simulink library "sm_flex_body_lib"  (R2016b)
settings: Solver=VariableStepAuto  StartTime=0.0  StopTime=10.0  RelTol=1e-3
values from neighbouring files (symbols this model uses):
  frameBody = splitBodyProps    [sm_flex_body_lib_fei_configure_beam.m]
undefined symbols (not defined in the file or in its folder): frameGraphic, X, Y, Z
undefined symbols (not defined in the file): beam_color, beam_opacity, beam_wall, beam_width, beamLink, brot_beamx, brot_beamy, brot_beamz, btra_beamx, elem_length, Extr_Data_Box, krot_beamx, krot_beamy, krot_beamz, ktra_beamx, rho, tau
libraries: sm_flex_body_lib x26, sm_lib x25, nesl_utility x24
(part 2 of 2)

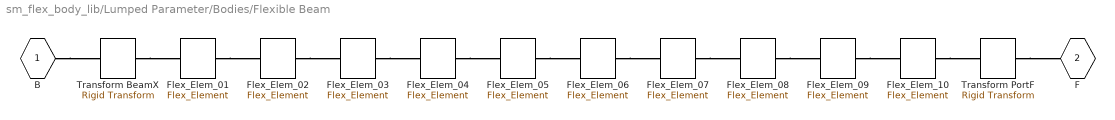
== system sm_flex_body_lib/Lumped Parameter/Bodies/Flexible Beam ==
  Flex_Elem_01 : sm_flex_body_lib/Lumped Parameter/Bodies/Flex_Element  be_length=elem_length  rho=rho  be_color=beam_color  be_opacity=beam_opacity  krot_beamz_elem=krot_beamz  brot_beamz_elem=brot_beamz  krot_beamy_elem=krot_beamy  brot_beamy_elem=brot_beamy  krot_beamx_elem=krot_beamx  brot_beamx_elem=brot_beamx  ktra_beamx_elem=ktra_beamx  btra_beamx_elem=btra_beamx  radio_flextype_elem=Rotation: Z
  Flex_Elem_02 : sm_flex_body_lib/Lumped Parameter/Bodies/Flex_Element  be_length=elem_length  rho=rho  be_color=beam_color  be_opacity=beam_opacity  krot_beamz_elem=krot_beamz  brot_beamz_elem=brot_beamz  krot_beamy_elem=krot_beamy  brot_beamy_elem=brot_beamy  krot_beamx_elem=krot_beamx  brot_beamx_elem=brot_beamx  ktra_beamx_elem=ktra_beamx  btra_beamx_elem=btra_beamx  radio_flextype_elem=Rotation: Z
  Flex_Elem_03 : sm_flex_body_lib/Lumped Parameter/Bodies/Flex_Element  be_length=elem_length  rho=rho  be_color=beam_color  be_opacity=beam_opacity  krot_beamz_elem=krot_beamz  brot_beamz_elem=brot_beamz  krot_beamy_elem=krot_beamy  brot_beamy_elem=brot_beamy  krot_beamx_elem=krot_beamx  brot_beamx_elem=brot_beamx  ktra_beamx_elem=ktra_beamx  btra_beamx_elem=btra_beamx  radio_flextype_elem=Rotation: Z
  Flex_Elem_04 : sm_flex_body_lib/Lumped Parameter/Bodies/Flex_Element  be_length=elem_length  rho=rho  be_color=beam_color  be_opacity=beam_opacity  krot_beamz_elem=krot_beamz  brot_beamz_elem=brot_beamz  krot_beamy_elem=krot_beamy  brot_beamy_elem=brot_beamy  krot_beamx_elem=krot_beamx  brot_beamx_elem=brot_beamx  ktra_beamx_elem=ktra_beamx  btra_beamx_elem=btra_beamx  radio_flextype_elem=Rotation: Z
  Flex_Elem_05 : sm_flex_body_lib/Lumped Parameter/Bodies/Flex_Element  be_length=elem_length  rho=rho  be_color=beam_color  be_opacity=beam_opacity  krot_beamz_elem=krot_beamz  brot_beamz_elem=brot_beamz  krot_beamy_elem=krot_beamy  brot_beamy_elem=brot_beamy  krot_beamx_elem=krot_beamx  brot_beamx_elem=brot_beamx  ktra_beamx_elem=ktra_beamx  btra_beamx_elem=btra_beamx  radio_flextype_elem=Rotation: Z
  Flex_Elem_06 : sm_flex_body_lib/Lumped Parameter/Bodies/Flex_Element  be_length=elem_length  rho=rho  be_color=beam_color  be_opacity=beam_opacity  krot_beamz_elem=krot_beamz  brot_beamz_elem=brot_beamz  krot_beamy_elem=krot_beamy  brot_beamy_elem=brot_beamy  krot_beamx_elem=krot_beamx  brot_beamx_elem=brot_beamx  ktra_beamx_elem=ktra_beamx  btra_beamx_elem=btra_beamx  radio_flextype_elem=Rotation: Z
  Flex_Elem_07 : sm_flex_body_lib/Lumped Parameter/Bodies/Flex_Element  be_length=elem_length  rho=rho  be_color=beam_color  be_opacity=beam_opacity  krot_beamz_elem=krot_beamz  brot_beamz_elem=brot_beamz  krot_beamy_elem=krot_beamy  brot_beamy_elem=brot_beamy  krot_beamx_elem=krot_beamx  brot_beamx_elem=brot_beamx  ktra_beamx_elem=ktra_beamx  btra_beamx_elem=btra_beamx  radio_flextype_elem=Rotation: Z
  Flex_Elem_08 : sm_flex_body_lib/Lumped Parameter/Bodies/Flex_Element  be_length=elem_length  rho=rho  be_color=beam_color  be_opacity=beam_opacity  krot_beamz_elem=krot_beamz  brot_beamz_elem=brot_beamz  krot_beamy_elem=krot_beamy  brot_beamy_elem=brot_beamy  krot_beamx_elem=krot_beamx  brot_beamx_elem=brot_beamx  ktra_beamx_elem=ktra_beamx  btra_beamx_elem=btra_beamx  radio_flextype_elem=Rotation: Z
  Flex_Elem_09 : sm_flex_body_lib/Lumped Parameter/Bodies/Flex_Element  be_length=elem_length  rho=rho  be_color=beam_color  be_opacity=beam_opacity  krot_beamz_elem=krot_beamz  brot_beamz_elem=brot_beamz  krot_beamy_elem=krot_beamy  brot_beamy_elem=brot_beamy  krot_beamx_elem=krot_beamx  brot_beamx_elem=brot_beamx  ktra_beamx_elem=ktra_beamx  btra_beamx_elem=btra_beamx  radio_flextype_elem=Rotation: Z
  Flex_Elem_10 : sm_flex_body_lib/Lumped Parameter/Bodies/Flex_Element  be_length=elem_length  rho=rho  be_color=beam_color  be_opacity=beam_opacity  krot_beamz_elem=krot_beamz  brot_beamz_elem=brot_beamz  krot_beamy_elem=krot_beamy  brot_beamy_elem=brot_beamy  krot_beamx_elem=krot_beamx  brot_beamx_elem=brot_beamx  ktra_beamx_elem=ktra_beamx  btra_beamx_elem=btra_beamx  radio_flextype_elem=Rotation: Z
  Transform BeamX : sm_lib/Frames and Transforms/Rigid Transform  TranslationMethod=StandardAxis  TranslationStandardOffset=0  TranslationLengthUnit=m  TranslationStandardAxis=+Z  TranslationCartesianOffset=[0 0 0]  TranslationROffset=0  TranslationROffsetUnits=m  TranslationZOffset=0  TranslationZOffsetUnits=m  TranslationThetaOffset=0  TranslationThetaOffsetUnits=deg  RotationMethod=StandardAxis  RotationAngleUnits=deg  RotationStandardAxis=+Y  RotationAngle=90  RotationArbitraryAxis=[0 0 1]  FollAlignAxisA=+X  BaseAlignAxisA=+Y  FollAlignAxisB=+Y  BaseAlignAxisB=+Z  RotationSequenceAxes=FollowerAxes  RotationSequence=XYX  RotationSequenceAngles=[0 0 0]  RotationSequenceAnglesUnits=deg  RotationMatrix=[1 0 0; 0 1 0; 0 0 1]
  Transform PortF : sm_lib/Frames and Transforms/Rigid Transform  TranslationMethod=None  TranslationStandardOffset=0  TranslationLengthUnit=m  TranslationStandardAxis=+Z  TranslationCartesianOffset=[0 0 0]  TranslationROffset=0  TranslationROffsetUnits=m  TranslationZOffset=0  TranslationZOffsetUnits=m  TranslationThetaOffset=0  TranslationThetaOffsetUnits=deg  RotationMethod=StandardAxis  RotationAngleUnits=deg  RotationStandardAxis=+Y  RotationAngle=-90  RotationArbitraryAxis=[0 0 1]  FollAlignAxisA=+X  BaseAlignAxisA=+Y  FollAlignAxisB=+Y  BaseAlignAxisB=+Z  RotationSequenceAxes=FollowerAxes  RotationSequence=XYX  RotationSequenceAngles=[0 0 0]  RotationSequenceAnglesUnits=deg  RotationMatrix=[1 0 0; 0 1 0; 0 0 1]
  B : PMIOPort  Port=1  Side=Left
  F : PMIOPort  Port=2  Side=Right
  connections:
  B/RConn1 -- Transform BeamX/LConn1
  Transform BeamX/RConn1 -- Flex_Elem_01/LConn1
  Flex_Elem_01/RConn1 -- Flex_Elem_02/LConn1
  Flex_Elem_02/RConn1 -- Flex_Elem_03/LConn1
  Flex_Elem_03/RConn1 -- Flex_Elem_04/LConn1
  Flex_Elem_04/RConn1 -- Flex_Elem_05/LConn1
  Flex_Elem_05/RConn1 -- Flex_Elem_06/LConn1
  Flex_Elem_06/RConn1 -- Flex_Elem_07/LConn1
  Flex_Elem_07/RConn1 -- Flex_Elem_08/LConn1
  Flex_Elem_08/RConn1 -- Flex_Elem_09/LConn1
  Flex_Elem_09/RConn1 -- Flex_Elem_10/LConn1
  Flex_Elem_10/RConn1 -- Transform PortF/LConn1
  Transform PortF/RConn1 -- F/RConn1

== system sm_flex_body_lib/FE Import/Bodies/Body 3 Frames/Routing Forces ==
  In1 : Inport
  Demux : Demux  Outputs=6*ones(1,3)
  F1 : Outport
  F2 : Outport  Port=2
  F3 : Outport  Port=3
  wires:
  Demux/2 -> F2/1
  In1/1 -> Demux/1
  Demux/1 -> F1/1
  Demux/3 -> F3/1

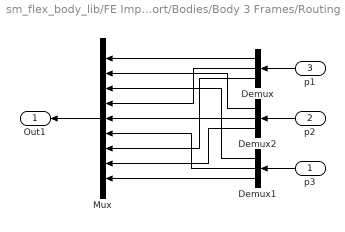
== system sm_flex_body_lib/FE Import/Bodies/Body 3 Frames/Routing pva ==
  p3 : Inport
  p2 : Inport  Port=2
  p1 : Inport  Port=3
  Demux : Demux  Outputs=3
  Demux1 : Demux  Outputs=3
  Demux2 : Demux  Outputs=3
  Mux : Mux  Inputs=9
  Out1 : Outport
  wires:
  Demux2/1 -> Mux/2
  Demux2/2 -> Mux/5
  Demux2/3 -> Mux/8
  p2/1 -> Demux2/1
  Demux1/3 -> Mux/9
  Demux/3 -> Mux/7
  Demux1/2 -> Mux/6
  Demux/2 -> Mux/4
  Demux1/1 -> Mux/3
  Demux/1 -> Mux/1
  p3/1 -> Demux1/1
  Mux/1 -> Out1/1
  p1/1 -> Demux/1

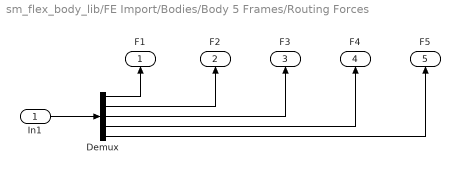
== system sm_flex_body_lib/FE Import/Bodies/Body 5 Frames/Routing Forces ==
  In1 : Inport
  Demux : Demux  Outputs=6*ones(1,5)
  F1 : Outport
  F2 : Outport  Port=2
  F3 : Outport  Port=3
  F4 : Outport  Port=4
  F5 : Outport  Port=5
  wires:
  Demux/3 -> F3/1
  Demux/1 -> F1/1
  In1/1 -> Demux/1
  Demux/2 -> F2/1
  Demux/4 -> F4/1
  Demux/5 -> F5/1

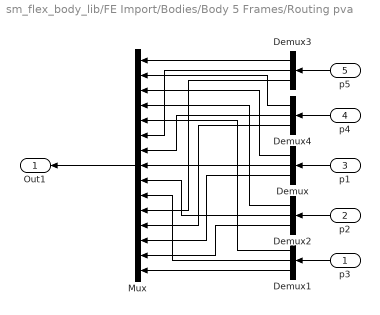
== system sm_flex_body_lib/FE Import/Bodies/Body 5 Frames/Routing pva ==
  p3 : Inport
  p2 : Inport  Port=2
  p1 : Inport  Port=3
  p4 : Inport  Port=4
  p5 : Inport  Port=5
  Demux{,1..4} (5 alike) : Demux  Outputs=3
  Mux : Mux  Inputs=15
  Out1 : Outport
  wires:
  p1/1 -> Demux/1
  Mux/1 -> Out1/1
  p3/1 -> Demux1/1
  p2/1 -> Demux2/1
  p5/1 -> Demux3/1
  Demux3/1 -> Mux/1
  Demux4/1 -> Mux/2
  Demux/1 -> Mux/3
  Demux2/1 -> Mux/4
  Demux1/1 -> Mux/5
  Demux3/2 -> Mux/6
  Demux4/2 -> Mux/7
  Demux/2 -> Mux/8
  Demux2/2 -> Mux/9
  Demux1/2 -> Mux/10
  Demux3/3 -> Mux/11
  Demux4/3 -> Mux/12
  Demux/3 -> Mux/13
  Demux2/3 -> Mux/14
  Demux1/3 -> Mux/15
  p4/1 -> Demux4/1

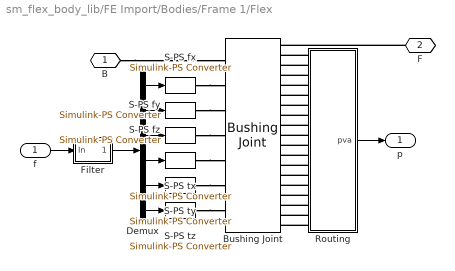
== system sm_flex_body_lib/FE Import/Bodies/Frame 1/Flex ==
  f : Inport
  Bushing Joint : sm_lib/Joints/Bushing Joint  SenseConstraintForce=off  SenseConstraintForceX=off  SenseConstraintForceY=off  SenseConstraintForceZ=off  SenseConstraintTorque=off  SenseConstraintTorqueX=off  SenseConstraintTorqueY=off  SenseConstraintTorqueZ=off  SenseTotalForce=off  SenseTotalForceX=off  SenseTotalForceY=off  SenseTotalForceZ=off  SenseTotalTorque=off  SenseTotalTorqueX=off  SenseTotalTorqueY=off  SenseTotalTorqueZ=off  CompositeWrenchDir=FollowerOnBase  CompositeWrenchFrame=BaseFrame  PxEquilibriumPosition=0  PxEquilibriumPositionUnits=m  PxSpringStiffness=0  PxSpringStiffnessUnits=N/m  PxDampingCoefficient=0  PxDampingCoefficientUnits=N/(m/s)  PxTorqueActuationMode=InputTorque  PxMotionActuationMode=ComputedMotion  PxSensePosition=on  PxSenseVelocity=on  PxSenseAcceleration=on  PxSenseTorqueForce=off  PxPositionTargetSpecify=off  PxPositionTargetPriority=High  PxPositionTargetValue=0  PxPositionTargetValueUnits=m  PxVelocityTargetSpecify=off  PxVelocityTargetPriority=High  PxVelocityTargetValue=0  PxVelocityTargetValueUnits=m/s  PyEquilibriumPosition=0  PyEquilibriumPositionUnits=m  PySpringStiffness=0  PySpringStiffnessUnits=N/m  PyDampingCoefficient=0  PyDampingCoefficientUnits=N/(m/s)  PyTorqueActuationMode=InputTorque  PyMotionActuationMode=ComputedMotion  PySensePosition=on  PySenseVelocity=on  PySenseAcceleration=on  PySenseTorqueForce=off  PyPositionTargetSpecify=off  PyPositionTargetPriority=High  PyPositionTargetValue=0  PyPositionTargetValueUnits=m  PyVelocityTargetSpecify=off  PyVelocityTargetPriority=High  PyVelocityTargetValue=0  PyVelocityTargetValueUnits=m/s  PzEquilibriumPosition=0  PzEquilibriumPositionUnits=m  PzSpringStiffness=0  PzSpringStiffnessUnits=N/m  PzDampingCoefficient=0  PzDampingCoefficientUnits=N/(m/s)  PzTorqueActuationMode=InputTorque  PzMotionActuationMode=ComputedMotion  PzSensePosition=on  PzSenseVelocity=on  PzSenseAcceleration=on  PzSenseTorqueForce=off  PzPositionTargetSpecify=off  PzPositionTargetPriority=High  PzPositionTargetValue=0  PzPositionTargetValueUnits=m  PzVelocityTargetSpecify=off  PzVelocityTargetPriority=High  PzVelocityTargetValue=0  PzVelocityTargetValueUnits=m/s  RxEquilibriumPosition=0  RxEquilibriumPositionUnits=deg  RxSpringStiffness=0  RxSpringStiffnessUnits=N*m/deg  RxDampingCoefficient=0  RxDampingCoefficientUnits=N*m/(deg/s)  RxTorqueActuationMode=InputTorque  RxMotionActuationMode=ComputedMotion  RxSensePosition=on  RxSenseVelocity=on  RxSenseAcceleration=on  RxSenseTorqueForce=off  RxPositionTargetSpecify=off  RxPositionTargetPriority=High  RxPositionTargetValue=0  RxPositionTargetValueUnits=deg  RxVelocityTargetSpecify=off  RxVelocityTargetPriority=High  RxVelocityTargetValue=0  RxVelocityTargetValueUnits=deg/s  RyEquilibriumPosition=0  RyEquilibriumPositionUnits=deg  RySpringStiffness=0  RySpringStiffnessUnits=N*m/deg  RyDampingCoefficient=0  RyDampingCoefficientUnits=N*m/(deg/s)  RyTorqueActuationMode=InputTorque  RyMotionActuationMode=ComputedMotion  RySensePosition=on  RySenseVelocity=on  RySenseAcceleration=on  RySenseTorqueForce=off  RyPositionTargetSpecify=off  RyPositionTargetPriority=High  RyPositionTargetValue=0  RyPositionTargetValueUnits=deg  RyVelocityTargetSpecify=off  RyVelocityTargetPriority=High  RyVelocityTargetValue=0  RyVelocityTargetValueUnits=deg/s  RzEquilibriumPosition=0  RzEquilibriumPositionUnits=deg  RzSpringStiffness=0  RzSpringStiffnessUnits=N*m/deg  RzDampingCoefficient=0  RzDampingCoefficientUnits=N*m/(deg/s)  RzTorqueActuationMode=InputTorque  RzMotionActuationMode=ComputedMotion  RzSensePosition=on  RzSenseVelocity=on  RzSenseAcceleration=on  RzSenseTorqueForce=off  RzPositionTargetSpecify=off  RzPositionTargetPriority=High  RzPositionTargetValue=0  RzPositionTargetValueUnits=deg  RzVelocityTargetSpecify=off  RzVelocityTargetPriority=High  RzVelocityTargetValue=0  RzVelocityTargetValueUnits=deg/s
  Demux : Demux  Outputs=6
  Filter : Subsystem  mask(First-order lag supporting vector signals){b=tau, x_initial=0}
      mask prompts: b "Filter time constant"; x_initial "Initial output"
      mask help: Models a lag of the form 1/(b*s+1) where s is the Laplace operator.
  Routing : Subsystem
  S-PS fx : nesl_utility/Simulink-PS Converter  PhysicalDomain=network_engine_domain  SubClassName=ps_input  LeftPortType=input  RightPortType=output  PseudoPeriodic=off  Frequencies=[]  NoiseDistribution=none  NoiseParameters=[]  Unit=N  AffineConversion=off  InputFiltering=off  SimscapeFilterOrder=1  InputFilterTimeConstant=0.001  UdotUserProvided=1
  S-PS fy : nesl_utility/Simulink-PS Converter  PhysicalDomain=network_engine_domain  SubClassName=ps_input  LeftPortType=input  RightPortType=output  PseudoPeriodic=off  Frequencies=[]  NoiseDistribution=none  NoiseParameters=[]  Unit=N  AffineConversion=off  InputFiltering=off  SimscapeFilterOrder=1  InputFilterTimeConstant=0.001  UdotUserProvided=1
  S-PS fz : nesl_utility/Simulink-PS Converter  PhysicalDomain=network_engine_domain  SubClassName=ps_input  LeftPortType=input  RightPortType=output  PseudoPeriodic=off  Frequencies=[]  NoiseDistribution=none  NoiseParameters=[]  Unit=N  AffineConversion=off  InputFiltering=off  SimscapeFilterOrder=1  InputFilterTimeConstant=0.001  UdotUserProvided=1
  S-PS tx : nesl_utility/Simulink-PS Converter  PhysicalDomain=network_engine_domain  SubClassName=ps_input  LeftPortType=input  RightPortType=output  PseudoPeriodic=off  Frequencies=[]  NoiseDistribution=none  NoiseParameters=[]  Unit=N*m  AffineConversion=off  InputFiltering=off  SimscapeFilterOrder=1  InputFilterTimeConstant=0.001  UdotUserProvided=1
  S-PS ty : nesl_utility/Simulink-PS Converter  PhysicalDomain=network_engine_domain  SubClassName=ps_input  LeftPortType=input  RightPortType=output  PseudoPeriodic=off  Frequencies=[]  NoiseDistribution=none  NoiseParameters=[]  Unit=N*m  AffineConversion=off  InputFiltering=off  SimscapeFilterOrder=1  InputFilterTimeConstant=0.001  UdotUserProvided=1
  S-PS tz : nesl_utility/Simulink-PS Converter  PhysicalDomain=network_engine_domain  SubClassName=ps_input  LeftPortType=input  RightPortType=output  PseudoPeriodic=off  Frequencies=[]  NoiseDistribution=none  NoiseParameters=[]  Unit=N*m  AffineConversion=off  InputFiltering=off  SimscapeFilterOrder=1  InputFilterTimeConstant=0.001  UdotUserProvided=1
  B : PMIOPort  Port=1  Side=Left
  F : PMIOPort  Port=2  Side=Right
  p : Outport
  wires:
  Routing/1(pva) -> p/1
  Demux/1 -> S-PS fx/1
  Demux/2 -> S-PS fy/1
  Demux/3 -> S-PS fz/1
  Demux/4 -> S-PS tx/1
  Demux/5 -> S-PS ty/1
  Demux/6 -> S-PS tz/1
  f/1 -> Filter/1(In)
  Filter/1(Out) -> Demux/1
  connections:
  Routing/LConn18 -- Bushing Joint/RConn19
  Routing/LConn17 -- Bushing Joint/RConn18
  Routing/LConn16 -- Bushing Joint/RConn17
  Routing/LConn15 -- Bushing Joint/RConn16
  Routing/LConn14 -- Bushing Joint/RConn15
  Routing/LConn13 -- Bushing Joint/RConn14
  Routing/LConn12 -- Bushing Joint/RConn13
  Routing/LConn11 -- Bushing Joint/RConn12
  Routing/LConn10 -- Bushing Joint/RConn11
  Routing/LConn9 -- Bushing Joint/RConn10
  Routing/LConn8 -- Bushing Joint/RConn9
  Routing/LConn7 -- Bushing Joint/RConn8
  Routing/LConn6 -- Bushing Joint/RConn7
  Routing/LConn5 -- Bushing Joint/RConn6
  Routing/LConn4 -- Bushing Joint/RConn5
  Routing/LConn3 -- Bushing Joint/RConn4
  Routing/LConn2 -- Bushing Joint/RConn3
  Routing/LConn1 -- Bushing Joint/RConn2
  B/RConn1 -- Bushing Joint/LConn1
  F/RConn1 -- Bushing Joint/RConn1
  S-PS fx/RConn1 -- Bushing Joint/LConn2
  S-PS fy/RConn1 -- Bushing Joint/LConn3
  S-PS fz/RConn1 -- Bushing Joint/LConn4
  S-PS tx/RConn1 -- Bushing Joint/LConn5
  S-PS ty/RConn1 -- Bushing Joint/LConn6
  S-PS tz/RConn1 -- Bushing Joint/LConn7

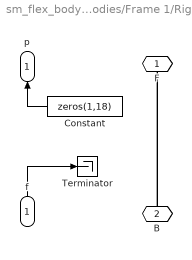
== system sm_flex_body_lib/FE Import/Bodies/Frame 1/Rigid ==
  f : Inport
  Constant : Constant  Value=zeros(1,18)
  Terminator : Terminator
  F : PMIOPort  Port=1  Side=Right
  B : PMIOPort  Port=2  Side=Left
  p : Outport
  wires:
  f/1 -> Terminator/1
  Constant/1 -> p/1
  connections:
  B/RConn1 -- F/RConn1

== system sm_flex_body_lib/FE Import/Bodies/Frame 1/Flex/Filter ==
  In : Inport
  Gain : Gain  Gain=1./b
  Integrator : Integrator  InitialCondition=x_initial.*b
  Sum : Sum  Inputs=|+-  SaturateOnIntegerOverflow=on  InputSameDT=on  OutDataTypeStr=Inherit: Same as first input
  Out : Outport
  wires:
  Gain/1 -> Out/1, Sum/2
  Integrator/1 -> Gain/1
  In/1 -> Sum/1
  Sum/1 -> Integrator/1

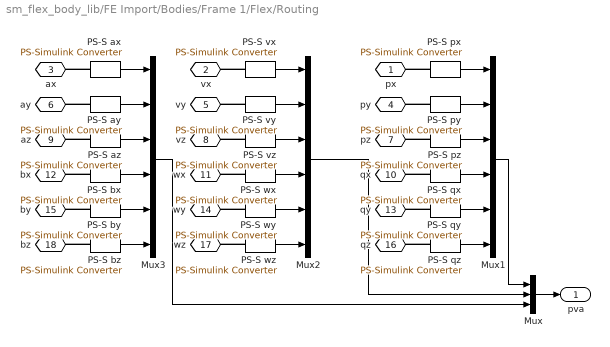
== system sm_flex_body_lib/FE Import/Bodies/Frame 1/Flex/Routing ==
  Mux : Mux  Inputs=3
  Mux1 : Mux  Inputs=6
  Mux2 : Mux  Inputs=6
  Mux3 : Mux  Inputs=6
  PS-S ax : nesl_utility/PS-Simulink Converter  PhysicalDomain=network_engine_domain  SubClassName=ps_output  LeftPortType=input  RightPortType=output  PseudoPeriodic=off  Frequencies=[]  Unit=m/s^2  AffineConversion=off
  PS-S ay : nesl_utility/PS-Simulink Converter  PhysicalDomain=network_engine_domain  SubClassName=ps_output  LeftPortType=input  RightPortType=output  PseudoPeriodic=off  Frequencies=[]  Unit=m/s^2  AffineConversion=off
  PS-S az : nesl_utility/PS-Simulink Converter  PhysicalDomain=network_engine_domain  SubClassName=ps_output  LeftPortType=input  RightPortType=output  PseudoPeriodic=off  Frequencies=[]  Unit=m/s^2  AffineConversion=off
  PS-S bx : nesl_utility/PS-Simulink Converter  PhysicalDomain=network_engine_domain  SubClassName=ps_output  LeftPortType=input  RightPortType=output  PseudoPeriodic=off  Frequencies=[]  Unit=rad/s^2  AffineConversion=off
  PS-S by : nesl_utility/PS-Simulink Converter  PhysicalDomain=network_engine_domain  SubClassName=ps_output  LeftPortType=input  RightPortType=output  PseudoPeriodic=off  Frequencies=[]  Unit=rad/s^2  AffineConversion=off
  PS-S bz : nesl_utility/PS-Simulink Converter  PhysicalDomain=network_engine_domain  SubClassName=ps_output  LeftPortType=input  RightPortType=output  PseudoPeriodic=off  Frequencies=[]  Unit=rad/s^2  AffineConversion=off
  PS-S px : nesl_utility/PS-Simulink Converter  PhysicalDomain=network_engine_domain  SubClassName=ps_output  LeftPortType=input  RightPortType=output  PseudoPeriodic=off  Frequencies=[]  Unit=m  AffineConversion=off
  PS-S py : nesl_utility/PS-Simulink Converter  PhysicalDomain=network_engine_domain  SubClassName=ps_output  LeftPortType=input  RightPortType=output  PseudoPeriodic=off  Frequencies=[]  Unit=m  AffineConversion=off
  PS-S pz : nesl_utility/PS-Simulink Converter  PhysicalDomain=network_engine_domain  SubClassName=ps_output  LeftPortType=input  RightPortType=output  PseudoPeriodic=off  Frequencies=[]  Unit=m  AffineConversion=off
  PS-S qx : nesl_utility/PS-Simulink Converter  PhysicalDomain=network_engine_domain  SubClassName=ps_output  LeftPortType=input  RightPortType=output  PseudoPeriodic=off  Frequencies=[]  Unit=rad  AffineConversion=off
  PS-S qy : nesl_utility/PS-Simulink Converter  PhysicalDomain=network_engine_domain  SubClassName=ps_output  LeftPortType=input  RightPortType=output  PseudoPeriodic=off  Frequencies=[]  Unit=rad  AffineConversion=off
  PS-S qz : nesl_utility/PS-Simulink Converter  PhysicalDomain=network_engine_domain  SubClassName=ps_output  LeftPortType=input  RightPortType=output  PseudoPeriodic=off  Frequencies=[]  Unit=rad  AffineConversion=off
  PS-S vx : nesl_utility/PS-Simulink Converter  PhysicalDomain=network_engine_domain  SubClassName=ps_output  LeftPortType=input  RightPortType=output  PseudoPeriodic=off  Frequencies=[]  Unit=m/s  AffineConversion=off
  PS-S vy : nesl_utility/PS-Simulink Converter  PhysicalDomain=network_engine_domain  SubClassName=ps_output  LeftPortType=input  RightPortType=output  PseudoPeriodic=off  Frequencies=[]  Unit=m/s  AffineConversion=off
  PS-S vz : nesl_utility/PS-Simulink Converter  PhysicalDomain=network_engine_domain  SubClassName=ps_output  LeftPortType=input  RightPortType=output  PseudoPeriodic=off  Frequencies=[]  Unit=m/s  AffineConversion=off
  PS-S wx : nesl_utility/PS-Simulink Converter  PhysicalDomain=network_engine_domain  SubClassName=ps_output  LeftPortType=input  RightPortType=output  PseudoPeriodic=off  Frequencies=[]  Unit=rad/s  AffineConversion=off
  PS-S wy : nesl_utility/PS-Simulink Converter  PhysicalDomain=network_engine_domain  SubClassName=ps_output  LeftPortType=input  RightPortType=output  PseudoPeriodic=off  Frequencies=[]  Unit=rad/s  AffineConversion=off
  PS-S wz : nesl_utility/PS-Simulink Converter  PhysicalDomain=network_engine_domain  SubClassName=ps_output  LeftPortType=input  RightPortType=output  PseudoPeriodic=off  Frequencies=[]  Unit=rad/s  AffineConversion=off
  px : PMIOPort  Port=1  Side=Left
  vx : PMIOPort  Port=2  Side=Left
  ax : PMIOPort  Port=3  Side=Left
  py : PMIOPort  Port=4  Side=Left
  vy : PMIOPort  Port=5  Side=Left
  ay : PMIOPort  Port=6  Side=Left
  pz : PMIOPort  Port=7  Side=Left
  vz : PMIOPort  Port=8  Side=Left
  az : PMIOPort  Port=9  Side=Left
  qx : PMIOPort  Port=10  Side=Left
  wx : PMIOPort  Port=11  Side=Left
  bx : PMIOPort  Port=12  Side=Left
  qy : PMIOPort  Port=13  Side=Left
  wy : PMIOPort  Port=14  Side=Left
  by : PMIOPort  Port=15  Side=Left
  qz : PMIOPort  Port=16  Side=Left
  wz : PMIOPort  Port=17  Side=Left
  bz : PMIOPort  Port=18  Side=Left
  pva : Outport
  wires:
  Mux/1 -> pva/1
  Mux3/1 -> Mux/3
  PS-S px/1 -> Mux1/1
  PS-S pz/1 -> Mux1/3
  PS-S vx/1 -> Mux2/1
  PS-S wx/1 -> Mux2/4
  Mux2/1 -> Mux/2
  PS-S vz/1 -> Mux2/3
  PS-S qz/1 -> Mux1/6
  PS-S qy/1 -> Mux1/5
  PS-S qx/1 -> Mux1/4
  PS-S vy/1 -> Mux2/2
  PS-S wz/1 -> Mux2/6
  PS-S wy/1 -> Mux2/5
  PS-S py/1 -> Mux1/2
  Mux1/1 -> Mux/1
  PS-S ax/1 -> Mux3/1
  PS-S by/1 -> Mux3/5
  PS-S bz/1 -> Mux3/6
  PS-S ay/1 -> Mux3/2
  PS-S az/1 -> Mux3/3
  PS-S bx/1 -> Mux3/4
  connections:
  PS-S pz/LConn1 -- pz/RConn1
  PS-S px/LConn1 -- px/RConn1
  PS-S wy/LConn1 -- wy/RConn1
  PS-S by/LConn1 -- by/RConn1
  PS-S bz/LConn1 -- bz/RConn1
  PS-S qy/LConn1 -- qy/RConn1
  PS-S ax/LConn1 -- ax/RConn1
  PS-S qz/LConn1 -- qz/RConn1
  PS-S vx/LConn1 -- vx/RConn1
  PS-S vy/LConn1 -- vy/RConn1
  PS-S wz/LConn1 -- wz/RConn1
  PS-S az/LConn1 -- az/RConn1
  PS-S bx/LConn1 -- bx/RConn1
  PS-S ay/LConn1 -- ay/RConn1
  PS-S wx/LConn1 -- wx/RConn1
  PS-S py/LConn1 -- py/RConn1
  PS-S qx/LConn1 -- qx/RConn1
  PS-S vz/LConn1 -- vz/RConn1
